simulink model "IMUData"  (R2024a)
settings: Solver=FixedStepAuto  StartTime=0.0  StopTime=100  FixedStep=.01  RelTol=1e-3  EnableMultiTasking=on
undefined symbols (not defined in the file or in its folder): CR, LF
libraries: instrumentseriallib x3, hdlsllib x1
settings Model: ExtModeTrigDuration=2  Creator=juanandrespelaezb  LastModifiedBy=juanandrespelaezb
settings SolverCC: AutoInsertRateTranBlk=on
settings OptimizationCC: EnhancedBackFolding=on  PassReuseOutputArgsAs=Individual arguments  ZeroExternalMemoryAtStartup=off  ZeroInternalMemoryAtStartup=off  MaxStackSize=64  OptimizeBlockOrder=speed  DifferentSizesBufferReuse=on  OptimizationCustomize=off  EfficientTunableParamExpr=on
settings DebuggingCC: ParameterTunabilityLossMsg=error
settings HardwareCC: ProdBitPerInt=16  ProdBitPerPointer=16  ProdBitPerSizeT=16  ProdBitPerPtrDiffT=16  ProdLargestAtomicFloat=None  ProdWordSize=8  ProdHWDeviceType=Atmel->AVR  UseEmbeddedCoderFeatures=off  UseSimulinkCoderFeatures=off
settings SFSimCC: MATLABDynamicMemAlloc=off
settings RTWCC: Description=Embedded Coder  SystemTargetFile=ert.tlc  HardwareBoard=Arduino Mega 2560  TemplateMakefile=ert_default_tmf  Toolchain=Arduino AVR  BuildConfiguration=Faster Runs
settings CodeAppCC: ForceParamTrailComments=on  IgnoreCustomStorageClasses=off  OperatorAnnotations=on  SimulinkDataObjDesc=on  SFDataObjDesc=on  InsertBlockDesc=on
settings ERTTargetCC: SupportContinuousTime=on  SupportNonInlinedSFcns=on  SupportVariableSizeSignals=on  ExtModeTransport=3  ExtModeStaticAlloc=on  ExtModeAutomaticAllocSize=off  ExtModeStaticAllocSize=2048  ExtModeMexFile=ext_xcp  ExtModeIntrfLevel=Level2 - Open

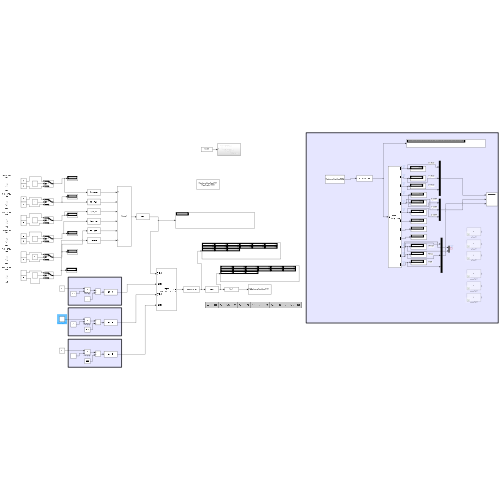
[thumbnail: Simulink's stored preview of the top-level diagram]
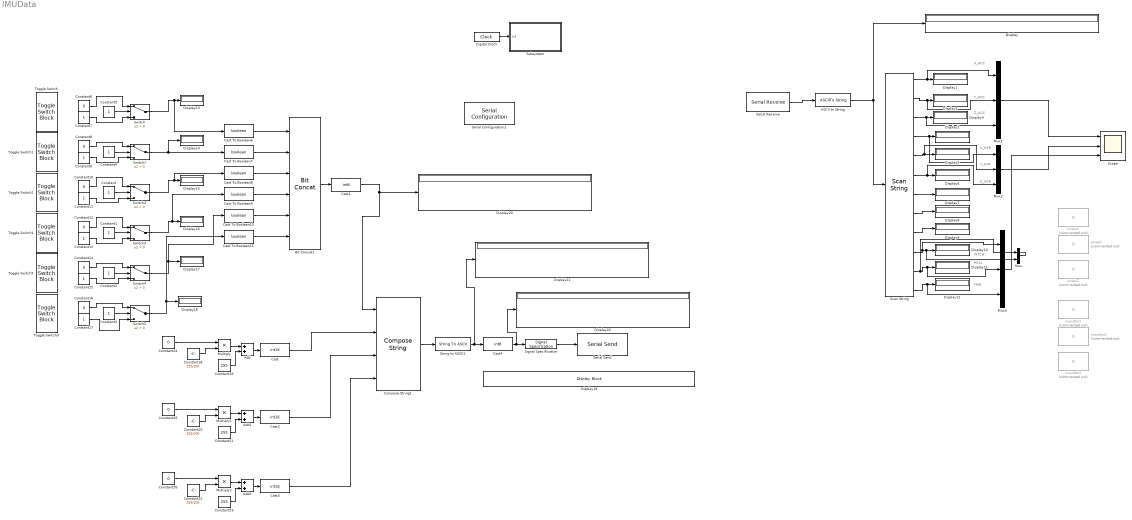
== system IMUData ==
  note: ROLL
  note: Z_GYR
  note: PITCH
  note: YAW
  note: Y_GYR
  note: X_GYR
  note: Z_ACC
  note: Y_ACC
  note: X_ACC
  ASCII to String : ASCIIToString
  Add : Sum
  Add1 : Sum
  Add2 : Sum
  Bit Concat1 : hdlsllib/Logic and Bit Operations/Bit Concat  numInputs=6
  Cast : DataTypeConversion  OutDataTypeStr=int16  SaturateOnIntegerOverflow=off  RndMeth=Floor
  Cast To Boolean{6..11} (6 alike) : DataTypeConversion  OutDataTypeStr=boolean  SaturateOnIntegerOverflow=off  RndMeth=Floor
  Cast1 : DataTypeConversion  OutDataTypeStr=int8  SaturateOnIntegerOverflow=off  RndMeth=Floor
  Cast2 : DataTypeConversion  OutDataTypeStr=int16  SaturateOnIntegerOverflow=off  RndMeth=Floor
  Cast3 : DataTypeConversion  OutDataTypeStr=int16  SaturateOnIntegerOverflow=off  RndMeth=Floor
  Cast4 : DataTypeConversion  OutDataTypeStr=int8  SaturateOnIntegerOverflow=off  RndMeth=Floor
  Compose String1 : ComposeString  Format="\"%02d;%03d;%03d;%03d\\n\""
  Constant{,1..5,7,9,11,13,15,17} (12 alike) : Constant
  Constant{6,8,10,12,14,16,24..26} (9 alike) : Constant  Value=0
  Constant18 : Constant  Value=255/100
  Constant19 : Constant  Value=255
  Constant20 : Constant  Value=255/100
  Constant21 : Constant  Value=255
  Constant22 : Constant  Value=255/100
  Constant23 : Constant  Value=255
  Digital Clock : DigitalClock
  Display{,1..18,20..22} (22 alike) : Display
  Display19 : DisplayBlock  LabelPosition=Hide  Format=long  Transparency=1
  Multiply : Product
  Multiply1 : Product
  Multiply2 : Product
  Mux : Mux  Inputs=2
  Mux1 : Mux  Inputs=3
  Mux2 : Mux  Inputs=3
  Mux3 : Mux  Inputs=3
  Scan String : ScanString  Format="\"%f,%f,%f,%f,%f,%f,%f,%f,%f,%f,%f,%f\""
  Scope : Scope  NumInputPorts=3
  Serial Configuration1 : instrumentseriallib/Serial Configuration  Priority=-200000  PortSel=/dev/cu.usbmodem2101  Port=/dev/cu.usbmodem2101  ComPort=/dev/cu.usbmodem2101  BaudRate=9600  DataBits=8  Parity=none  StopBits=1  ByteOrder=little-endian  FlowControl=none  Timeout=10  SimulateUsing=Interpreted execution  BlockInModel=on  aMode=1
  Serial Receive : instrumentseriallib/Serial Receive  PortSel=/dev/cu.usbmodem2101  Port=/dev/cu.usbmodem2101  ComPort=/dev/cu.usbmodem2101  DataType=uint8  SaveDataType=uint8  ToggleHeader=off  Header=[]  ToggleDataSize=on  DataSize=76  ToggleTerminator=on  Terminator=CR/LF ('\r\n')  CustomTerminator=[]  InputFormat=Column major  EnableBlockingMode=on  ActionDataUnavailable=Output last received value  ActionWhenDataUnavailable=Output last received value  CustomValue=300  SampleTime=.01  SimulateUsing=Interpreted execution  BlockInModel=on  aMode=1
  Serial Send : instrumentseriallib/Serial Send  PortSel=/dev/cu.usbmodem2101  Port=/dev/cu.usbmodem2101  ComPort=/dev/cu.usbmodem2101  Header=[]  Terminator=<none>  CustomTerminator=[]  EnableBlockingMode=on  SimulateUsing=Interpreted execution  BlockInModel=on  aMode=1
  Signal Specification : SignalSpecification  SampleTime=.1
      settings: LockScale=on
  String to ASCII1 : StringToASCII  OutputVectorSize=15
  Subsystem : Subsystem
  Switch{,1..5} (6 alike) : Switch  Criteria=u2 > Threshold  SaturateOnIntegerOverflow=off  InputSameDT=off
  Toggle Switch{,1..5} (6 alike) : ToggleSwitchBlock
      settings: Values={{'Off', 'On'}, [0 1]}
  massBal1 : Constant  Commented=on  Value=0
  massBal2 : Constant  Commented=on  Value=0
  massBal3 : Constant  Commented=on  Value=0
  wheelX : Constant  Commented=on  Value=0
  wheelY : Constant  Commented=on  Value=0
  wheelZ : Constant  Commented=on  Value=0
  wires:
  Mux/1 -> ?
  Scan String/2 -> Mux1/2, Display3/1
  ASCII to String/1 -> Display/1, Scan String/1
  Scan String/7 -> Display7/1
  Scan String/1 -> Mux1/1, Display1/1
  Mux2/1 -> Scope/2
  Scan String/11 -> Mux/1, Mux3/2, Display11/1
  Mux1/1 -> Scope/1
  Scan String/6 -> Mux2/3, Display6/1
  Scan String/3 -> Mux1/3, Display4/1
  Scan String/5 -> Mux2/2, Display5/1
  Scan String/8 -> Display8/1
  Scan String/4 -> Mux2/1, Display2/1
  Scan String/9 -> Display9/1
  Scan String/12 -> Mux3/3, Display12/1
  Scan String/10 -> Mux3/1, Mux/2, Display10/1
  Digital Clock/1 -> Subsystem/1(In1)
  Serial Receive/1 -> ASCII to String/1
  Constant6/1 -> Switch/1
  Constant7/1 -> Switch/3
  Constant8/1 -> Switch1/1
  Constant9/1 -> Switch1/3
  Constant10/1 -> Switch2/1
  Constant11/1 -> Switch2/3
  Constant13/1 -> Switch3/3
  Constant12/1 -> Switch3/1
  Constant14/1 -> Switch4/1
  Constant15/1 -> Switch4/3
  Constant16/1 -> Switch5/1
  Constant17/1 -> Switch5/3
  Constant/1 -> Switch2/2
  Constant1/1 -> Switch3/2
  Constant2/1 -> Switch4/2
  Constant3/1 -> Switch5/2
  Constant4/1 -> Switch1/2
  Constant5/1 -> Switch/2
  Switch/1 -> Cast To Boolean6/1, Display13/1
  Switch1/1 -> Cast To Boolean7/1, Display14/1
  Switch2/1 -> Cast To Boolean8/1, Display15/1
  Switch3/1 -> Cast To Boolean9/1, Display16/1
  Switch4/1 -> Cast To Boolean10/1, Display17/1
  Switch5/1 -> Cast To Boolean11/1, Display18/1
  Cast To Boolean9/1 -> Bit Concat1/4
  Cast To Boolean7/1 -> Bit Concat1/2
  Cast To Boolean10/1 -> Bit Concat1/5
  Cast To Boolean6/1 -> Bit Concat1/1
  Cast To Boolean8/1 -> Bit Concat1/3
  Cast To Boolean11/1 -> Bit Concat1/6
  Bit Concat1/1 -> Cast1/1
  Cast1/1 -> Display20/1, Compose String1/1
  Cast2/1 -> Compose String1/3
  Constant21/1 -> Add1/2
  Constant19/1 -> Add/2
  Constant20/1 -> Multiply1/2
  Multiply1/1 -> Add1/1
  Constant18/1 -> Multiply/2
  Constant23/1 -> Add2/2
  Cast/1 -> Compose String1/2
  Add1/1 -> Cast2/1
  Cast3/1 -> Compose String1/4
  Add/1 -> Cast/1
  Multiply/1 -> Add/1
  Add2/1 -> Cast3/1
  Multiply2/1 -> Add2/1
  Constant22/1 -> Multiply2/2
  Constant26/1 -> Multiply2/1
  Constant25/1 -> Multiply1/1
  Constant24/1 -> Multiply/1
  Compose String1/1 -> String to ASCII1/1
  String to ASCII1/1 -> Display21/1, Cast4/1
  Cast4/1 -> Display22/1, Signal Specification/1
  Signal Specification/1 -> Serial Send/1
  Mux3/1 -> Scope/3

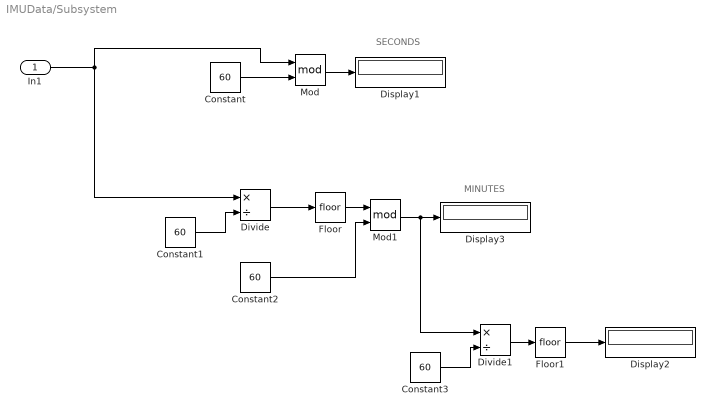
== system IMUData/Subsystem ==
  note: SECONDS
  note: MINUTES
  In1 : Inport
  Constant{,1..3} (4 alike) : Constant  Value=60
  Display1 : Display
  Display2 : Display
  Display3 : Display
  Divide : Product  Inputs=*/
  Divide1 : Product  Inputs=*/
  Floor : Rounding
  Floor1 : Rounding
  Mod : Math  Operator=mod  SignedPower=on
  Mod1 : Math  Operator=mod  SignedPower=on
  wires:
  Constant/1 -> Mod/2
  Mod/1 -> Display1/1
  In1/1 -> Divide/1, Mod/1
  Constant1/1 -> Divide/2
  Divide/1 -> Floor/1
  Floor/1 -> Mod1/1
  Constant2/1 -> Mod1/2
  Mod1/1 -> Divide1/1, Display3/1
  Constant3/1 -> Divide1/2
  Divide1/1 -> Floor1/1
  Floor1/1 -> Display2/1
